simulink model "doc_hamming"  (R2014a)
settings: Solver=VariableStepDiscrete  StartTime=0.0  StopTime=inf  RelTol=1e-3
undefined symbols (not defined in the file or in its folder): gfprimfd
libraries: commblkcod2 x8, commrandsrc2 x4, commsink2 x4, commchan3 x3, commdigbbndpm3 x2, commutil2 x2, simulink x1
settings Model: Creator=The MathWorks Inc.
settings DataIOCC: SignalLoggingSaveFormat=ModelDataLogs
settings OptimizationCC: BlockReduction=off  BooleanDataType=off  ExpressionDepthLimit=2147483647
settings DebuggingCC: SaveWithParameterizedLinksMsg=none  UnderspecifiedInitializationDetection=Classic  SignalResolutionControl=TryResolveAllWithWarning  SolverPrmCheckMsg=none  MultiTaskDSMMsg=warning  MultiTaskCondExecSysMsg=none  FcnCallInpInsideContextMsg=UseLocalSettings  StateNameClashWarn=warning  StrictBusMsg=None
settings HardwareCC: TargetUnknown=on
settings RTWCC: IncludeERTFirstTime=on
settings GRTTargetCC: CombineOutputUpdateFcns=off  GRTInterface=on

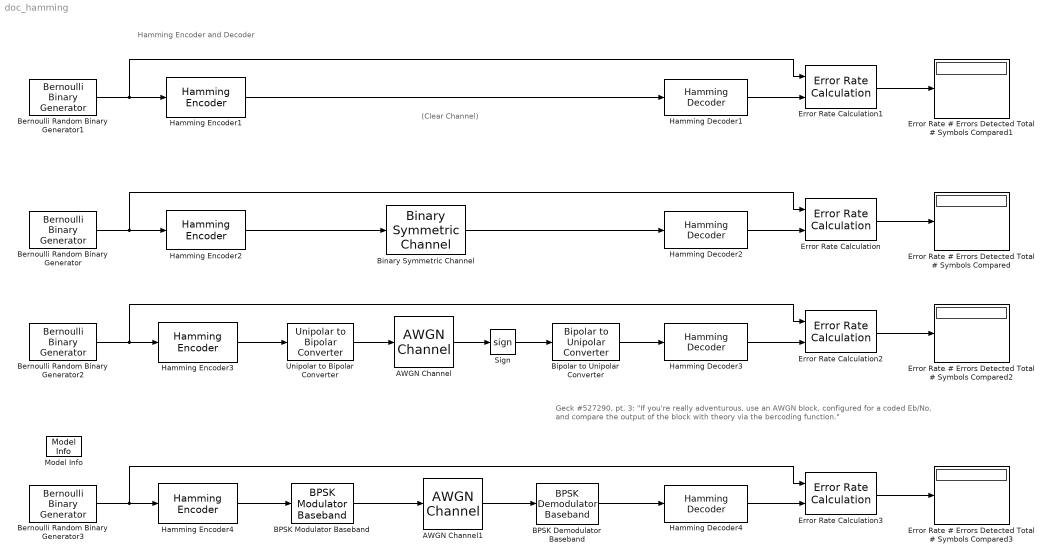
== system doc_hamming ==
  note: Hamming Encoder and Decoder
  note: (Clear Channel)
  note: Geck #527290, pt. 3: "If you're really adventurous, use an AWGN block, configured for a coded Eb/No, and compare the output of the block with theory via the bercoding function."
  AWGN Channel : commchan3/AWGN Channel  InputProcessing=Columns as channels (frame based)  seed=67  noiseMode="Signal to noise ratio  (Eb/No)"  EbNodB=10+10*log10(4/7)  EsNodB=10  SNRdB=10  bitsPerSym=1  Ps=1  Tsym=1  variance=1
  AWGN Channel1 : commchan3/AWGN Channel  InputProcessing=Columns as channels (frame based)  seed=67  noiseMode="Signal to noise ratio  (Eb/No)"  EbNodB=10+10*log10(4/7)  EsNodB=10  SNRdB=10  bitsPerSym=1  Ps=1  Tsym=1  variance=1
  BPSK Demodulator Baseband : commdigbbndpm3/BPSK Demodulator Baseband  Ph=0  DecType=Hard decision  VarSource=Dialog  Variance=1  outDtype=boolean  derotateFactorWordLen=16
  BPSK Modulator Baseband : commdigbbndpm3/BPSK Modulator Baseband  Ph=0  outDtype=double  outWordLen=16  outUDDataType=sfix(16)  outFracLenMode=Best precision  outFracLen=15
  Bernoulli Random Binary Generator{,1..3} (4 alike) : commrandsrc2/Bernoulli Binary Generator  P=.5  seed=92748  Ts=1  frameBased=on  sampPerFrame=4  orient=off  outDataType=boolean
  Binary Symmetric Channel : commchan3/Binary Symmetric Channel  P=0.006  s=71  E=off  outDtype=boolean
  Bipolar to Unipolar Converter : commutil2/Bipolar to Unipolar Converter  M=2  polarity=Positive  dataType=boolean
  Error Rate # Errors Detected Total # Symbols Compared{,1..3} (4 alike) : Display
  Error Rate Calculation : commsink2/Error Rate Calculation  N=0  st_delay=0  cp_mode=Entire frame  subframe=[]  PMode=Port  WsName=ErrorVec  RsMode2=off  stop=off  numErr=100  maxBits=1e6
  Error Rate Calculation1 : commsink2/Error Rate Calculation  N=0  st_delay=0  cp_mode=Entire frame  subframe=[]  PMode=Port  WsName=ErrorVec  RsMode2=off  stop=off  numErr=100  maxBits=1e6
  Error Rate Calculation2 : commsink2/Error Rate Calculation  N=0  st_delay=0  cp_mode=Entire frame  subframe=[]  PMode=Port  WsName=ErrorVec  RsMode2=off  stop=off  numErr=100  maxBits=1e6
  Error Rate Calculation3 : commsink2/Error Rate Calculation  N=0  st_delay=0  cp_mode=Entire frame  subframe=[]  PMode=Port  WsName=ErrorVec  RsMode2=off  stop=on  numErr=100  maxBits=1e6
  Hamming Decoder{1..4} (4 alike) : commblkcod2/Hamming Decoder  n=7  k=gfprimfd(3,'min')
  Hamming Encoder{1..4} (4 alike) : commblkcod2/Hamming Encoder  n=7  k=gfprimfd(3,'min')
  Model Info : simulink/Model-Wide Utilities/Model Info  InitialBlockCM=None  BlockCM=none  Frame=on  DisplayStringWithTags=|  HorizontalTextAlignment=Center  LeftAlignmentValue=0.5  SourceBlockDiagram=doc_hamming  TagMaxNumber=20
      | Info
      | %<Description>
  Sign : Signum
  Unipolar to Bipolar Converter : commutil2/Unipolar to Bipolar Converter  M=2  polarity=Positive  dataType=double
  wires:
  Bernoulli Random Binary Generator/1 -> Error Rate Calculation/1, Hamming Encoder2/1
  Hamming Decoder2/1 -> Error Rate Calculation/2
  Error Rate Calculation/1 -> Error Rate # Errors Detected Total # Symbols Compared/1
  Hamming Encoder2/1 -> Binary Symmetric Channel/1
  Binary Symmetric Channel/1 -> Hamming Decoder2/1
  Bernoulli Random Binary Generator1/1 -> Hamming Encoder1/1, Error Rate Calculation1/1
  Hamming Decoder1/1 -> Error Rate Calculation1/2
  Error Rate Calculation1/1 -> Error Rate # Errors Detected Total # Symbols Compared1/1
  Hamming Encoder1/1 -> Hamming Decoder1/1
  Bernoulli Random Binary Generator2/1 -> Error Rate Calculation2/1, Hamming Encoder3/1
  Hamming Decoder3/1 -> Error Rate Calculation2/2
  Error Rate Calculation2/1 -> Error Rate # Errors Detected Total # Symbols Compared2/1
  Hamming Encoder3/1 -> Unipolar to Bipolar Converter/1
  Bipolar to Unipolar Converter/1 -> Hamming Decoder3/1
  Unipolar to Bipolar Converter/1 -> AWGN Channel/1
  AWGN Channel/1 -> Sign/1
  Bernoulli Random Binary Generator3/1 -> Hamming Encoder4/1, Error Rate Calculation3/1
  Hamming Decoder4/1 -> Error Rate Calculation3/2
  Error Rate Calculation3/1 -> Error Rate # Errors Detected Total # Symbols Compared3/1
  Hamming Encoder4/1 -> BPSK Modulator Baseband/1
  AWGN Channel1/1 -> BPSK Demodulator Baseband/1
  BPSK Demodulator Baseband/1 -> Hamming Decoder4/1
  BPSK Modulator Baseband/1 -> AWGN Channel1/1
  Sign/1 -> Bipolar to Unipolar Converter/1
